simulink library "HANcoder_STM32_Target"  (R2023a)
settings: Solver=ode45  StartTime=0.0  StopTime=10.0  RelTol=1e-3  EnableMultiTasking=on
libraries: simulink x3
(part 6 of 7)

== system HANcoder_STM32_Target/Olimexino STM32/Timer Outputs/Schedule Compare Event ==
  In1 : Inport
  In2 : Inport  Port=2
  Level-2 M-file S-Function : M-S-Function  FunctionName=sfcn_timeout_scheduleevent  Parameters=tsamp
  wires:
  In1/1 -> Level-2 M-file S-Function/1
  In2/1 -> Level-2 M-file S-Function/2

== system HANcoder_STM32_Target/Olimexino STM32/UART/UART init ==
  Level-2 M-file S-Function : M-S-Function  FunctionName=sfcn_uart_init
  Term1 : Terminator
  wires:
  Level-2 M-file S-Function/1 -> Term1/1

== system HANcoder_STM32_Target/Olimexino STM32/UART/UART receive ==
  Level-2 M-file S-Function : M-S-Function  FunctionName=sfcn_uart_receive  Parameters=tsamp
  Term1 : Terminator
  Out1 : Outport
  wires:
  Level-2 M-file S-Function/2 -> Term1/1
  Level-2 M-file S-Function/1 -> Out1/1

== system HANcoder_STM32_Target/Olimexino STM32/UART/UART receive buffer status ==
  Level-2 M-file S-Function : M-S-Function  FunctionName=sfcn_uart_receive_size  Parameters=tsamp
  Out1 : Outport
  wires:
  Level-2 M-file S-Function/1 -> Out1/1

== system HANcoder_STM32_Target/Olimexino STM32/UART/UART send ==
  In1 : Inport
  Level-2 M-file S-Function : M-S-Function  FunctionName=sfcn_uart_send  Parameters=tsamp
  Term1 : Terminator
  wires:
  In1/1 -> Level-2 M-file S-Function/1
  Level-2 M-file S-Function/1 -> Term1/1

== system HANcoder_STM32_Target/Olimexino STM32/UDS/UDS Get Key ==
  S-Function : M-S-Function  FunctionName=sfcn_uds_get_key  Parameters=tsamp
  Out1 : Outport
  wires:
  S-Function/1 -> Out1/1

== system HANcoder_STM32_Target/Olimexino STM32/UDS/UDS Get Seed ==
  S-Function : M-S-Function  FunctionName=sfcn_uds_get_seed  Parameters=tsamp
  Out1 : Outport
  wires:
  S-Function/1 -> Out1/1

== system HANcoder_STM32_Target/Olimexino STM32/UDS/UDS Get Seed Event ==
  S-Function : S-Function  FunctionName=sfcn_uds_get_seed_event  SFunctionDeploymentMode=off  EnableBusSupport=off
  Out1 : Outport
  wires:
  S-Function/1 -> Out1/1

== system HANcoder_STM32_Target/Olimexino STM32/UDS/UDS Init ==
  S-Function : M-S-Function  FunctionName=sfcn_uds_init

== system HANcoder_STM32_Target/Olimexino STM32/UDS/UDS Set Key Verfied ==
  In1 : Inport
  S-Function : M-S-Function  FunctionName=sfcn_uds_set_key_verified  Parameters=tsamp
  wires:
  In1/1 -> S-Function/1

== system HANcoder_STM32_Target/Olimexino STM32/UDS/UDS Set Seed ==
  In1 : Inport
  S-Function : M-S-Function  FunctionName=sfcn_uds_set_seed  Parameters=tsamp
  wires:
  In1/1 -> S-Function/1

== system HANcoder_STM32_Target/Olimexino STM32/UDS/UDS Verify Key Event ==
  S-Function : S-Function  FunctionName=sfcn_uds_verify_key_event  SFunctionDeploymentMode=off  EnableBusSupport=off
  Out1 : Outport
  wires:
  S-Function/1 -> Out1/1

== system HANcoder_STM32_Target/STM32-E407/Analog Inputs/Analog Input ==
  Level-2 M-file S-Function : M-S-Function  FunctionName=sfcn_analog_in  Parameters=tsamp, pinID
  Out1 : Outport
  wires:
  Level-2 M-file S-Function/1 -> Out1/1

== system HANcoder_STM32_Target/STM32-E407/Analog Outputs/Analog Output ==
  In1 : Inport
  Data Type Conversion : DataTypeConversion  OutDataTypeStr=uint16  SaturateOnIntegerOverflow=off  RndMeth=Floor
  Level-2 M-file S-Function : M-S-Function  FunctionName=sfcn_analog_out  Parameters=tsamp, pinID
  Saturation : Saturate  UpperLimit=4095  LowerLimit=0
  wires:
  Saturation/1 -> Level-2 M-file S-Function/1
  Data Type Conversion/1 -> Saturation/1
  In1/1 -> Data Type Conversion/1

== system HANcoder_STM32_Target/STM32-E407/CAN/CAN ==
  CAN receive : Subsystem  Tag=HANcoder_TARGET_STM32_E407  mask(CAN receive){canBus=CAN 1, outputNumber=1, dataType=uint8, byteOrder=off, tsamp=-1}
      mask prompts: canBus "CAN channel"; outputNumber "Output ports"; dataType "Output datatype"; byteOrder "Byte order: Checked = MSB first, unchecked = LSB first."; tsamp "Sample time"
      mask help:
      | Function
      | ==========
      | Receive the newest message from the specified CAN channel.
      |
      | Parameters
      | ==========
      | CAN channel:             The CAN channel to send the message on.
      | Output ports:             The amount of output ports
      | Output datatype:       The datatype of the output ports
      | Byte order:                 Select MSB or LSB first
      | Sample time:              -1 or divisible by base sample time [seconds]
      |
      | Input
      | ==========
      | Port 1:                       CAN ID(uint32) in hexadecimal ie: hex2dec('0a')
      |
      | Output
      | ==========
      | Port 1:                       Checks for new message(int8)
      | Port 2..9                     Message data
      mask init:
      | sfcn_can_receive_mcb(canBus, outputNumber, dataType, byteOrder)
      settings: MoveFcn=drawLogos
      mask Help: web('sfcn_can_receive.html');
      mask TypeOptions canBus: CAN 1 | CAN 2
      mask TypeOptions dataType: int8 | uint8 | int16 | uint16 | int32 | uint32 | boolean
      mask Display:
      | fprintf('Receive on\nCAN %x', canBus);
      | port_label('output', 1, 'new');
      | port_label('input', 1, 'ID');patch([75 81 81],[8 14 2],[1 0 0]);patch([83 83 89],[14 2 8],[0 0 0.35]);
  CAN receive packed : Subsystem  Tag=HANcoder_TARGET_STM32_E407  mask(CAN receive packed){canBus=CAN 1, canID=hex2dec('80'), tsamp=-1}
      mask prompts: canBus "CAN channel"; canID "Can ID (in hex)"; tsamp "Sample time"
      mask help:
      | Function
      | ==========
      | Receive the newest message from the specified CAN channel, packed in a CAN message signal.
      | The first output checks the receiving of new data.
      |
      | CAN channel: The specified CAN channel will be used to receive the message on.
      |
      | CAN ID (in hex): Only the message with the specified CAN identifier (ID) is received. The ID is written in hexadecimal format, ie: hex2dec('0A')
      |
      | PS. No data is unpacked by the 'CAN Unpack' block when the data output is directly connected to a terminator (an example, placing a *1 'Gain' in between will solve this).
      mask init:
      | sfcn_can_receive_packed_mcb(canBus, canID)
      settings: MoveFcn=drawLogos
      mask Help: web('sfcn_can_receive_packed.html');
      mask TypeOptions canBus: CAN 1 | CAN 2
      mask Display: fprintf('Receive packed CAN\nmessage on CAN %x\nID %xh', canBus, canID);patch([95 101 101],[8 14 2],[1 0 0]);patch([103 103 109],[14 2 8],[0 0 0.35]);
  CAN send : Subsystem  Tag=HANcoder_TARGET_STM32_E407  mask(CAN send){canBus=CAN 1, frameType=Standard (11 bit), inputNumber=8, dataType=uint8, byteOrder=on, tsamp=-1}
      mask prompts: canBus "CAN channel"; frameType "Identifier type"; inputNumber "Input ports"; dataType "Input datatype"; byteOrder "Byte order: Checked = MSB first, unchecked = LSB first."; tsamp "Sample time"
      mask help:
      | Function
      | ==========
      | Send a message on the CAN channel.
      |
      | Parameters
      | ==========
      | CAN channel:           The CAN channel to send the message on.
      | Identifier type:         normal or extended ID's
      | Input ports:              The amount of input ports
      | Input datatype:        The datatype of the input ports
      | Byte order:               Select MSB or LSB first
      | Sample time:            -1 or divisible by base sample time [seconds]
      |
      | Input
      | ==========
      | Port 1:                   CAN ID(uint32) in hexadecimal ie: hex2dec('0a')
      | Port 2..9                CAN message data
      mask init:
      | sfcn_can_send_mcb(canBus, frameType, inputNumber, dataType, byteOrder)
      settings: MoveFcn=drawLogos
      mask Help: web('sfcn_can_send.html');
      mask TypeOptions canBus: CAN 1 | CAN 2
      mask TypeOptions frameType: Standard (11 bit) | Extended (29 bit)
      mask TypeOptions dataType: int8 | uint8 | int16 | uint16 | int32 | uint32 | boolean
      mask Display:
      | fprintf('Send on\nCAN %x', canBus);
      | port_label('input', 1, 'ID');patch([65 71 71],[8 14 2],[1 0 0]);patch([73 73 79],[14 2 8],[0 0 0.35]);
  CAN send packed : Subsystem  Tag=HANcoder_TARGET_STM32_E407  mask(CAN send packed){canBus=CAN 1, tsamp=-1}
      mask prompts: canBus "CAN channel"; tsamp "Sample time"
      mask help:
      | Function
      | ==========
      | Send a packed CAN message on the specified CAN channel.
      |
      | CAN channel: The specified CAN channel will be used to send the message on.
      |
      | The CAN ID, identifier type and formatting of the data is included in the packed CAN message.
      mask init:
      | sfcn_can_send_packed_mcb(canBus)
      settings: MoveFcn=drawLogos
      mask Help: web('sfcn_can_send_packed.html');
      mask TypeOptions canBus: CAN 1 | CAN 2
      mask Display: fprintf('Send packed CAN\n message on CAN %x', canBus);patch([95 101 101],[8 14 2],[1 0 0]);patch([103 103 109],[14 2 8],[0 0 0.35]);

== system HANcoder_STM32_Target/STM32-E407/CAN/CANopenNode ==
  CANopenNode Init : Subsystem  Tag=HANcoder_TARGET_STM32_E407  mask(CANopenNode Init){channel=CAN 1}
      mask prompts: channel "CAN channel"
      mask help:
      | Function
      | ==========
      | Initializes the CANopenNode stack for the particular CAN channel.
      |
      | CAN channel: The specified CAN channel will be used by the communication stack.
      mask init:
      | sfcn_can_canopennode_init_mcb(channel)
      settings: MoveFcn=drawLogos
      mask Help: web('sfcn_can_canopennode_init.html');
      mask TypeOptions channel: CAN 1 | CAN 2
      mask Display: fprintf('CANopenNode\n Init on CAN %d', channel);patch([95 101 101],[8 14 2],[1 0 0]);patch([103 103 109],[14 2 8],[0 0 0.35]);
  CANopenNode OD Read : Subsystem  Tag=HANcoder_TARGET_STM32_E407  mask(CANopenNode OD Read){index=hex2dec('6200'), subIndex=1, dataType=uint8, tsamp=-1}
      mask prompts: index "OD index"; subIndex "OD subindex"; dataType "OD data type"; tsamp "Sample time"
      mask help:
      | Function
      | ==========
      | Reads a data value from the internal object dictionary.
      |
      | OD Index: Index of the object dictionary to read from.
      | OD Subindex: Subindex of the object dictionary to read from.
      | OD Data type: Data type of the object dictionary to read from.
      mask init:
      | sfcn_can_canopennode_od_read_mcb(index, subIndex, dataType)
      settings: MoveFcn=drawLogos
      mask Help: web('sfcn_can_canopennode_od_read.html');
      mask TypeOptions dataType: int8 | uint8 | int16 | uint16 | int32 | uint32
      mask Display: fprintf('CANopenNode\n OD Read\nindex: 0x%x\nsubindex: %d', index, subIndex');patch([95 101 101],[8 14 2],[1 0 0]);patch([103 103 109],[14 2 8],[0 0 0.35]);
  CANopenNode OD Write : Subsystem  Tag=HANcoder_TARGET_STM32_E407  mask(CANopenNode OD Write){index=hex2dec('6000'), subIndex=1, dataType=uint8, tsamp=-1}
      mask prompts: index "OD index"; subIndex "OD subindex"; dataType "OD data type"; tsamp "Sample time"
      mask help:
      | Function
      | ==========
      | Writes a data value to the internal object dictionary.
      |
      | OD Index: Index of the object dictionary to write to.
      | OD Subindex: Subindex of the object dictionary to write to.
      | OD Data type: Data type of the object dictionary to write to.
      mask init:
      | sfcn_can_canopennode_od_write_mcb(index, subIndex, dataType)
      settings: MoveFcn=drawLogos
      mask Help: web('sfcn_can_canopennode_od_write.html');
      mask TypeOptions dataType: int8 | uint8 | int16 | uint16 | int32 | uint32
      mask Display: fprintf('CANopenNode\n OD Write\nindex: 0x%x\nsubindex: %d', index, subIndex);patch([95 101 101],[8 14 2],[1 0 0]);patch([103 103 109],[14 2 8],[0 0 0.35]);

== system HANcoder_STM32_Target/STM32-E407/Digital Inputs/Digital Input ==
  Level-2 M-file S-Function : M-S-Function  FunctionName=sfcn_digital_in  Parameters=tsamp, pinID, config
  Out1 : Outport
  wires:
  Level-2 M-file S-Function/1 -> Out1/1

== system HANcoder_STM32_Target/STM32-E407/Digital Outputs/Digital Output ==
  In1 : Inport
  Level-2 M-file S-Function : M-S-Function  FunctionName=sfcn_digital_out  Parameters=tsamp, pinID, config
  wires:
  In1/1 -> Level-2 M-file S-Function/1

== system HANcoder_STM32_Target/STM32-E407/Error Handling/Clear errors ==
  Trigger : TriggerPort  VariantControl=(inherit)
  Level-2 M-file S-Function : M-S-Function  FunctionName=sfcn_controller_error_clearerrors  Parameters=eepromString

== system HANcoder_STM32_Target/STM32-E407/Error Handling/Delete error ==
  Trigger : TriggerPort  VariantControl=(inherit)
  Constant : Constant  OutDataTypeStr=uint8  SampleTime=-1
  Gnd1 : Ground
  Gnd2 : Ground
  Level-2 M-file S-Function : M-S-Function  FunctionName=sfcn_controller_error_deleteerror_in  Parameters=useInPorts, errorID, para
  wires:
  Constant/1 -> Level-2 M-file S-Function/3
  Gnd1/1 -> Level-2 M-file S-Function/1
  Gnd2/1 -> Level-2 M-file S-Function/2

== system HANcoder_STM32_Target/STM32-E407/Error Handling/Read active error ==
  In1 : Inport
  Level-2 M-file S-Function : M-S-Function  FunctionName=sfcn_controller_error_readerror  Parameters=tsamp
  numbers : Outport
  code : Outport  Port=2
  parameter : Outport  Port=3
  Xtimes : Outport  Port=4
  timestamp : Outport  Port=5
  wires:
  In1/1 -> Level-2 M-file S-Function/1
  Level-2 M-file S-Function/5 -> timestamp/1
  Level-2 M-file S-Function/4 -> Xtimes/1
  Level-2 M-file S-Function/3 -> parameter/1
  Level-2 M-file S-Function/2 -> code/1
  Level-2 M-file S-Function/1 -> numbers/1

== system HANcoder_STM32_Target/STM32-E407/Error Handling/Read stored error ==
  In1 : Inport
  Level-2 M-file S-Function : M-S-Function  FunctionName=sfcn_controller_error_readerror  Parameters=tsamp
  numbers : Outport
  code : Outport  Port=2
  parameter : Outport  Port=3
  Xtimes : Outport  Port=4
  timestamp : Outport  Port=5
  wires:
  Level-2 M-file S-Function/1 -> numbers/1
  Level-2 M-file S-Function/2 -> code/1
  Level-2 M-file S-Function/3 -> parameter/1
  Level-2 M-file S-Function/4 -> Xtimes/1
  Level-2 M-file S-Function/5 -> timestamp/1
  In1/1 -> Level-2 M-file S-Function/1

== system HANcoder_STM32_Target/STM32-E407/Error Handling/Search active error ==
  In1 : Inport
  In2 : Inport  Port=2
  Level-2 M-file S-Function : M-S-Function  FunctionName=sfcn_controller_error_searcherror  Parameters=tsamp
  occurrence : Outport
  timestamp : Outport  Port=2
  wires:
  Level-2 M-file S-Function/2 -> timestamp/1
  Level-2 M-file S-Function/1 -> occurrence/1
  In2/1 -> Level-2 M-file S-Function/2
  In1/1 -> Level-2 M-file S-Function/1

== system HANcoder_STM32_Target/STM32-E407/Error Handling/Search stored error ==
  In1 : Inport
  In2 : Inport  Port=2
  Level-2 M-file S-Function : M-S-Function  FunctionName=sfcn_controller_error_searcherror  Parameters=tsamp
  occurrence : Outport
  timestamp : Outport  Port=2
  wires:
  In1/1 -> Level-2 M-file S-Function/1
  In2/1 -> Level-2 M-file S-Function/2
  Level-2 M-file S-Function/1 -> occurrence/1
  Level-2 M-file S-Function/2 -> timestamp/1

== system HANcoder_STM32_Target/STM32-E407/Error Handling/Store error  ==
  Trigger : TriggerPort  VariantControl=(inherit)
  Gnd1 : Ground
  Gnd2 : Ground
  Level-2 M-file S-Function : M-S-Function  FunctionName=sfcn_controller_error_storeerror_in  Parameters=useInPorts, errorCode, parameter
  wires:
  Gnd2/1 -> Level-2 M-file S-Function/2
  Gnd1/1 -> Level-2 M-file S-Function/1

== system HANcoder_STM32_Target/STM32-E407/Error Handling/Total Errors ==
  Level-2 M-file S-Function : M-S-Function  FunctionName=sfcn_controller_error_totalerrors  Parameters=eepromString, tsamp
  Out1 : Outport
  Out2 : Outport  Port=2
  wires:
  Level-2 M-file S-Function/2 -> Out2/1
  Level-2 M-file S-Function/1 -> Out1/1

== system HANcoder_STM32_Target/STM32-E407/File Logger/File Logger Close ==
  Trigger : TriggerPort  VariantControl=(inherit)
  Level-2 M-file S-Function : M-S-Function  FunctionName=sfcn_filelogger_close

== system HANcoder_STM32_Target/STM32-E407/File Logger/File Logger Init ==
  (Re)start : TriggerPort  VariantControl=(inherit)
  Level-2 M-file S-Function : M-S-Function  FunctionName=sfcn_filelogger_init

== system HANcoder_STM32_Target/STM32-E407/File Logger/File Logger Signal ==
  In1 : Inport
  Level-2 M-file S-Function : M-S-Function  FunctionName=sfcn_filelogger_signal  Parameters=dataType
  wires:
  In1/1 -> Level-2 M-file S-Function/1

== system HANcoder_STM32_Target/STM32-E407/Memory/EEPROM ==
  Erase EEPROM : Subsystem  Tag=HANcoder_TARGET_STM32_E407  mask(Erase EEPROM){}
      mask help:
      | Function
      | ========
      | Erases all identifier values from EEPROM.
      |
      | Triggerport
      | ===========
      | Connect the port to a trigger source to execute the block only when necessary.
      mask init:
      | sfcn_eeprom_clear_mcb();
      settings: MoveFcn=drawLogos
      mask Display: fprintf('Erase EEPROM');patch([80 86 86],[8 14 2],[1 0 0]);patch([88 88 94],[14 2 8],[0 0 0.35]);
  Read from EEPROM : Subsystem  Tag=HANcoder_TARGET_STM32_E407  mask(Read from EEPROM){tsamp=-1}
      mask prompts: tsamp "Sample time"
      mask help:
      | Function
      | ========
      | Read a value from the specified EEPROM identifier.
      |
      | Inport
      | ==========
      | id:
      |   The EEPROM identifier. This input is of type UINT8 and can have a value
      |   between 0..255 to select one of the 256 supported application specific
      |   identifiers.
      |
      | Outport
      | =======
      | value:
      |   The value read from the EEPROM identifier. This output is of type UINT16.
      mask init:
      | sfcn_eeprom_read_mcb();
      settings: MoveFcn=drawLogos
      mask Display:
      | fprintf('Read from EEPROM');
      | port_label('input', 1, 'id');
      | port_label('output', 1, 'value');patch([150 156 156],[8 14 2],[1 0 0]);patch([158 158 164],[14 2 8],[0 0 0.35]);
  Save EEPROM : Subsystem  Tag=HANcoder_TARGET_STM32_E407  mask(Save EEPROM){}
      mask help:
      | Function
      | ========
      | The STM32 controller does not have dedicated EEPROM on-chip. All EEPROM
      | write, read and erase operations are therefore performed in a RAM buffer.
      | To make sure RAM buffer contents are still valid after a power-off, its
      | contents needs to be save in flash EEPROM, which is achieved with this
      | block. This is typically called during the software shutdown sequence,
      | right before power off.
      |
      | Triggerport
      | ===========
      | Connect the port to a trigger source to execute the block only when necessary.
      mask init:
      | sfcn_eeprom_save_mcb();
      settings: MoveFcn=drawLogos
      mask Display: fprintf('Save EEPROM');patch([80 86 86],[8 14 2],[1 0 0]);patch([88 88 94],[14 2 8],[0 0 0.35]);
  Write to EEPROM : Subsystem  Tag=HANcoder_TARGET_STM32_E407  mask(Write to EEPROM){tsamp=-1}
      mask prompts: tsamp "Sample time"
      mask help:
      | Function
      | ========
      | Write the value to the specified EEPROM identifier.
      |
      | Inport
      | ==========
      | id:
      |   The EEPROM identifier. This input is of type UINT8 and can have a value
      |   between 0..255 to select one of the 256 supported application specific
      |   identifiers.
      | value:
      |   The value to write to the EEPROM identifier. This input is of type UINT16.
      mask init:
      | sfcn_eeprom_write_mcb();
      settings: MoveFcn=drawLogos
      mask Display:
      | fprintf('Write to EEPROM');
      | port_label('input', 1, 'id');
      | port_label('input', 2, 'value');patch([150 156 156],[8 14 2],[1 0 0]);patch([158 158 164],[14 2 8],[0 0 0.35]);

== system HANcoder_STM32_Target/STM32-E407/PWM Outputs/PWM Duty Cycle ==
  In1 : Inport
  Level-2 M-file S-Function : M-S-Function  FunctionName=sfcn_pwmout_setduty  Parameters=tsamp
  wires:
  In1/1 -> Level-2 M-file S-Function/1

== system HANcoder_STM32_Target/STM32-E407/PWM Outputs/PWM Init ==
  S-Function : S-Function  FunctionName=sfcn_pwmout_init  SFunctionDeploymentMode=off  EnableBusSupport=off
  Term1 : Terminator
  wires:
  S-Function/1 -> Term1/1

== system HANcoder_STM32_Target/STM32-E407/Real-time Clock/Get Real-time Clock ==
  Level-2 M-file S-Function : M-S-Function  FunctionName=sfcn_get_rtc  Parameters=tsamp
  WeekDay : Outport
  Date : Outport  Port=2
  Month : Outport  Port=3
  Year : Outport  Port=4
  Hours : Outport  Port=5
  Minutes : Outport  Port=6
  Seconds : Outport  Port=7
  wires:
  Level-2 M-file S-Function/3 -> Month/1
  Level-2 M-file S-Function/6 -> Minutes/1
  Level-2 M-file S-Function/5 -> Hours/1
  Level-2 M-file S-Function/4 -> Year/1
  Level-2 M-file S-Function/1 -> WeekDay/1
  Level-2 M-file S-Function/7 -> Seconds/1
  Level-2 M-file S-Function/2 -> Date/1

== system HANcoder_STM32_Target/STM32-E407/Real-time Clock/Set Real-time Clock ==
  WeekDay : Inport
  Date : Inport  Port=2
  Month : Inport  Port=3
  Year : Inport  Port=4
  Hours : Inport  Port=5
  Minutes : Inport  Port=6
  Seconds : Inport  Port=7
  Trigger : TriggerPort  VariantControl=(inherit)  PortDimensions=1
  Level-2 M-file S-Function : M-S-Function  FunctionName=sfcn_set_rtc
  wires:
  WeekDay/1 -> Level-2 M-file S-Function/1
  Date/1 -> Level-2 M-file S-Function/2
  Month/1 -> Level-2 M-file S-Function/3
  Year/1 -> Level-2 M-file S-Function/4
  Hours/1 -> Level-2 M-file S-Function/5
  Minutes/1 -> Level-2 M-file S-Function/6
  Seconds/1 -> Level-2 M-file S-Function/7

== system HANcoder_STM32_Target/STM32-E407/SPI/SPI master init ==
  Level-2 M-file S-Function : M-S-Function  FunctionName=sfcn_spi_master_init

== system HANcoder_STM32_Target/STM32-E407/SPI/SPI master transfer ==
  In1 : Inport
  Level-2 M-file S-Function : M-S-Function  FunctionName=sfcn_spi_master_transfer  Parameters=tsamp
  Out1 : Outport
  wires:
  Level-2 M-file S-Function/1 -> Out1/1
  In1/1 -> Level-2 M-file S-Function/1

== system HANcoder_STM32_Target/STM32-E407/System Config/Base Sample Time config ==
  note: This constant and terminator block introduces the base sample time,
      | set in Base Sample Time config block, to the model. Blocks  with inherited [-1]
      | sample time wich are not connected to blocks with specifically set sample times
      | will use this value. This block also sets the fixed step time parameter in the Simulink Solver.
      | This works during initialization of simulation or build.
  Level-2 M-file S-Function : M-S-Function  FunctionName=sfcn_base_sample_time  Parameters=baseSampleTime, extraStack
  SampleTimeCrowBar : Constant  InitFcn=|  VectorParams1D=off  OutDataTypeStr=boolean  SampleTime=0.01
      | SampleTimeMiliSeconds = get_param(find_system(bdroot, 'LookUnderMasks', 'all', 'FollowLinks', 'off',  'Name', 'Base Sample Time config'), 'baseSampleTime');
      |                                                                                                                                                             
      | SampleTimeSeconds = str2num(SampleTimeMiliSeconds{1,1})/1000;                                                                                               
      |                                                                                                                                                             
      | set_param(bdroot, 'FixedStep', num2str(SampleTimeSeconds));                                                                                                 
      |                                                                                                                                                             
      | set_param(gcb, 'SampleTime', num2str(get_param(bdroot, 'FixedStep')));                                                                                      
      | clear SampleTimeSeconds SampleTimeMiliSeconds
  Terminator : Terminator
  wires:
  SampleTimeCrowBar/1 -> Terminator/1

== system HANcoder_STM32_Target/STM32-E407/System Config/Build settings ==

== system HANcoder_STM32_Target/STM32-E407/System Config/CAN config ==
  Level-2 M-file S-Function : M-S-Function  FunctionName=sfcn_can_config

== system HANcoder_STM32_Target/STM32-E407/System Config/Custom ID config ==
  Level-2 M-file S-Function : M-S-Function  RequirementInfo={}  FunctionName=sfcn_custom_version_config  Parameters=softID

== system HANcoder_STM32_Target/STM32-E407/System Config/Ethernet config ==
  Level-2 M-file S-Function : M-S-Function  FunctionName=sfcn_ethernet_config

== system HANcoder_STM32_Target/STM32-E407/System Config/FTP server config ==
  Level-2 M-file S-Function : M-S-Function  FunctionName=sfcn_ftp_server_config

== system HANcoder_STM32_Target/STM32-E407/System Config/XCP on CAN config ==
  Level-2 M-file S-Function : M-S-Function  RequirementInfo={} %GIDa_75ebdf1d_e085_4bd4_9cf7_36846954f0a6  FunctionName=sfcn_can_xcp_config  Parameters=canBus, croID, dtoID

== system HANcoder_STM32_Target/STM32-E407/System Config/XCP on TCP//IP config ==
  Level-2 M-file S-Function : M-S-Function  RequirementInfo={} %GIDa_75ebdf1d_e085_4bd4_9cf7_36846954f0a6  FunctionName=sfcn_tcpip_xcp_config  Parameters=port

== system HANcoder_STM32_Target/STM32-E407/System Config/XCP on USB config ==
  Level-2 M-file S-Function : M-S-Function  RequirementInfo={} %GIDa_75ebdf1d_e085_4bd4_9cf7_36846954f0a6  FunctionName=sfcn_usb_xcp_config

== system HANcoder_STM32_Target/STM32-E407/System Management/Enter Critical Section ==
  Level-2 M-file S-Function : M-S-Function  FunctionName=sfcn_critical_enter  Parameters=tsamp

== system HANcoder_STM32_Target/STM32-E407/System Management/Exit Critical Section ==
  Level-2 M-file S-Function : M-S-Function  FunctionName=sfcn_critical_exit  Parameters=tsamp

== system HANcoder_STM32_Target/STM32-E407/System Management/Get CPU load ==
  Level-2 M-file S-Function : M-S-Function  FunctionName=sfcn_controller_cpu_getload  Parameters=tsamp, mode
  Out1 : Outport
  wires:
  Level-2 M-file S-Function/1 -> Out1/1

== system HANcoder_STM32_Target/STM32-E407/System Management/Get free Heap ==
  Level-2 M-file S-Function : M-S-Function  FunctionName=sfcn_controller_getheap  Parameters=tsamp
  Out1 : Outport
  wires:
  Level-2 M-file S-Function/1 -> Out1/1

== system HANcoder_STM32_Target/STM32-E407/System Management/Get free Stack ==
  Level-2 M-file S-Function : M-S-Function  FunctionName=sfcn_controller_getstack  Parameters=tsamp, taskIdx
  Out1 : Outport
  wires:
  Level-2 M-file S-Function/1 -> Out1/1

== system HANcoder_STM32_Target/STM32-E407/System Management/Reset ECU ==
  Trigger : TriggerPort  VariantControl=(inherit)
  Level-2 M-file S-Function : M-S-Function  FunctionName=sfcn_controller_reset

== system HANcoder_STM32_Target/STM32-E407/Timer Inputs/Quadrature Encoder Get ==
  Data Type Conversion : DataTypeConversion  OutDataTypeStr=boolean  SaturateOnIntegerOverflow=off  RndMeth=Floor
  Detect Increase : simulink/Logic and Bit Operations/Detect Increase  vinit=0.0  OutDataTypeStr=uint8
  Gnd1 : Ground
  Level-2 M-file S-Function : M-S-Function  FunctionName=sfcn_quad_encoder_get  Parameters=tsamp, moduleID
  Out1 : Outport
  wires:
  Data Type Conversion/1 -> Level-2 M-file S-Function/1
  Detect Increase/1 -> Data Type Conversion/1
  Gnd1/1 -> Detect Increase/1
  Level-2 M-file S-Function/1 -> Out1/1

== system HANcoder_STM32_Target/STM32-E407/Timer Inputs/Timer Input Get ==
  Level-2 M-file S-Function : M-S-Function  FunctionName=sfcn_timein_get  Parameters=tsamp
  Out1 : Outport
  Out2 : Outport  Port=2
  Out3 : Outport  Port=3
  Out4 : Outport  Port=4
  Out5 : Outport  Port=5
  Out6 : Outport  Port=6
  Out7 : Outport  Port=7
  wires:
  Level-2 M-file S-Function/5 -> Out5/1
  Level-2 M-file S-Function/4 -> Out4/1
  Level-2 M-file S-Function/3 -> Out3/1
  Level-2 M-file S-Function/2 -> Out2/1
  Level-2 M-file S-Function/1 -> Out1/1
  Level-2 M-file S-Function/6 -> Out6/1
  Level-2 M-file S-Function/7 -> Out7/1

== system HANcoder_STM32_Target/STM32-E407/Timer Inputs/Timer Input IRQ ==
  S-Function : S-Function  FunctionName=sfcn_timein_irq  SFunctionDeploymentMode=off  EnableBusSupport=off
  Out1 : Outport
  wires:
  S-Function/1 -> Out1/1

== system HANcoder_STM32_Target/STM32-E407/Timer Outputs/Compare Event IRQ ==
  S-Function : S-Function  FunctionName=sfcn_timeout_event_irq  SFunctionDeploymentMode=off  EnableBusSupport=off
  Out1 : Outport
  wires:
  S-Function/1 -> Out1/1

== system HANcoder_STM32_Target/STM32-E407/Timer Outputs/Get Free Running Counter ==
  Level-2 M-file S-Function : M-S-Function  FunctionName=sfcn_timeout_getrunningcounter  Parameters=tsamp
  Out1 : Outport
  wires:
  Level-2 M-file S-Function/1 -> Out1/1

== system HANcoder_STM32_Target/STM32-E407/Timer Outputs/Get Last Event Counter ==
  Level-2 M-file S-Function : M-S-Function  FunctionName=sfcn_timeout_getlasteventcounter  Parameters=tsamp
  Out1 : Outport
  wires:
  Level-2 M-file S-Function/1 -> Out1/1

== system HANcoder_STM32_Target/STM32-E407/Timer Outputs/Output Compare Init ==
  S-Function : S-Function  FunctionName=sfcn_timeout_init  SFunctionDeploymentMode=off  EnableBusSupport=off
  Term1 : Terminator
  wires:
  S-Function/1 -> Term1/1

== system HANcoder_STM32_Target/STM32-E407/Timer Outputs/Reset Free Running Counter ==
  Trigger : TriggerPort  VariantControl=(inherit)
  Level-2 M-file S-Function : M-S-Function  FunctionName=sfcn_timeout_resetcounter

== system HANcoder_STM32_Target/STM32-E407/Timer Outputs/Schedule Compare Event ==
  In1 : Inport
  In2 : Inport  Port=2
  Level-2 M-file S-Function : M-S-Function  FunctionName=sfcn_timeout_scheduleevent  Parameters=tsamp
  wires:
  In1/1 -> Level-2 M-file S-Function/1
  In2/1 -> Level-2 M-file S-Function/2

== system HANcoder_STM32_Target/STM32-E407/UART/UART init ==
  Level-2 M-file S-Function : M-S-Function  FunctionName=sfcn_uart_init
  Term1 : Terminator
  wires:
  Level-2 M-file S-Function/1 -> Term1/1

== system HANcoder_STM32_Target/STM32-E407/UART/UART receive ==
  Level-2 M-file S-Function : M-S-Function  FunctionName=sfcn_uart_receive  Parameters=tsamp
  Term1 : Terminator
  Out1 : Outport
  wires:
  Level-2 M-file S-Function/1 -> Out1/1
  Level-2 M-file S-Function/2 -> Term1/1

== system HANcoder_STM32_Target/STM32-E407/UART/UART receive buffer status ==
  Level-2 M-file S-Function : M-S-Function  FunctionName=sfcn_uart_receive_size  Parameters=tsamp
  Out1 : Outport
  wires:
  Level-2 M-file S-Function/1 -> Out1/1

== system HANcoder_STM32_Target/STM32-E407/UART/UART send ==
  In1 : Inport
  Level-2 M-file S-Function : M-S-Function  FunctionName=sfcn_uart_send  Parameters=tsamp
  Term1 : Terminator
  wires:
  Level-2 M-file S-Function/1 -> Term1/1
  In1/1 -> Level-2 M-file S-Function/1

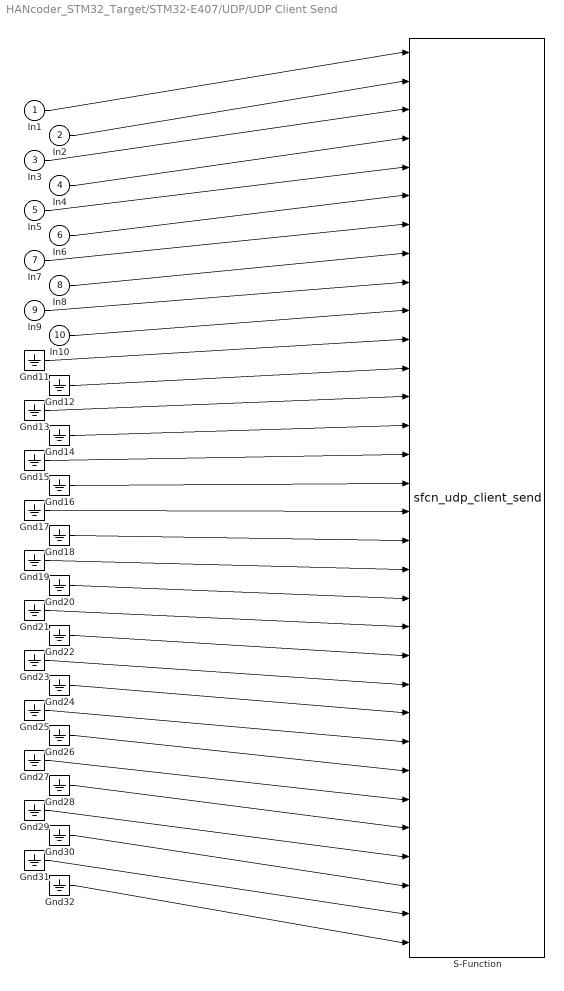
== system HANcoder_STM32_Target/STM32-E407/UDP/UDP Client Send ==
  In1 : Inport
  In2 : Inport  Port=2
  In3 : Inport  Port=3
  In4 : Inport  Port=4
  In5 : Inport  Port=5
  In6 : Inport  Port=6
  In7 : Inport  Port=7
  In8 : Inport  Port=8
  In9 : Inport  Port=9
  In10 : Inport  Port=10
  Gnd{11..32} (22 alike) : Ground
  S-Function : M-S-Function  FunctionName=sfcn_udp_client_send  Parameters=tsamp, dataType
  wires:
  In1/1 -> S-Function/1
  In2/1 -> S-Function/2
  In3/1 -> S-Function/3
  In4/1 -> S-Function/4
  In5/1 -> S-Function/5
  In6/1 -> S-Function/6
  In7/1 -> S-Function/7
  In8/1 -> S-Function/8
  In9/1 -> S-Function/9
  In10/1 -> S-Function/10
  Gnd11/1 -> S-Function/11
  Gnd12/1 -> S-Function/12
  Gnd13/1 -> S-Function/13
  Gnd14/1 -> S-Function/14
  Gnd15/1 -> S-Function/15
  Gnd16/1 -> S-Function/16
  Gnd17/1 -> S-Function/17
  Gnd18/1 -> S-Function/18
  Gnd19/1 -> S-Function/19
  Gnd20/1 -> S-Function/20
  Gnd21/1 -> S-Function/21
  Gnd22/1 -> S-Function/22
  Gnd23/1 -> S-Function/23
  Gnd24/1 -> S-Function/24
  Gnd25/1 -> S-Function/25
  Gnd26/1 -> S-Function/26
  Gnd27/1 -> S-Function/27
  Gnd28/1 -> S-Function/28
  Gnd29/1 -> S-Function/29
  Gnd30/1 -> S-Function/30
  Gnd31/1 -> S-Function/31
  Gnd32/1 -> S-Function/32

== system HANcoder_STM32_Target/STM32-E407/UDP/UDP Server Init ==
  S-Function : M-S-Function  FunctionName=sfcn_udp_server_init

== system HANcoder_STM32_Target/STM32-E407/UDP/UDP Server New Data Available ==
  S-Function : M-S-Function  FunctionName=sfcn_udp_server_new  Parameters=tsamp
  Out1 : Outport
  wires:
  S-Function/1 -> Out1/1

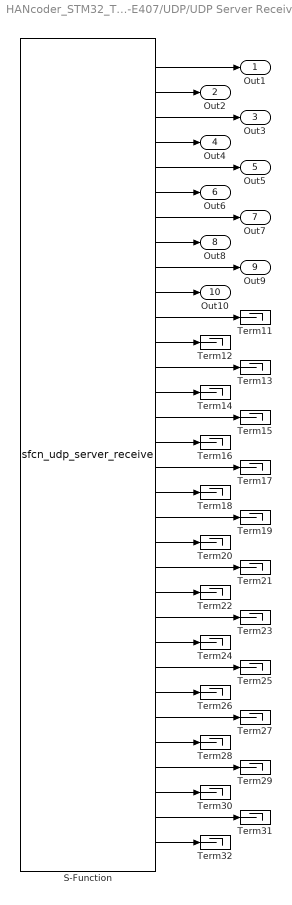
== system HANcoder_STM32_Target/STM32-E407/UDP/UDP Server Receive ==
  S-Function : M-S-Function  FunctionName=sfcn_udp_server_receive  Parameters=tsamp, dataType
  Term{11..32} (22 alike) : Terminator
  Out1 : Outport
  Out2 : Outport  Port=2
  Out3 : Outport  Port=3
  Out4 : Outport  Port=4
  Out5 : Outport  Port=5
  Out6 : Outport  Port=6
  Out7 : Outport  Port=7
  Out8 : Outport  Port=8
  Out9 : Outport  Port=9
  Out10 : Outport  Port=10
  wires:
  S-Function/1 -> Out1/1
  S-Function/2 -> Out2/1
  S-Function/3 -> Out3/1
  S-Function/4 -> Out4/1
  S-Function/5 -> Out5/1
  S-Function/6 -> Out6/1
  S-Function/7 -> Out7/1
  S-Function/8 -> Out8/1
  S-Function/9 -> Out9/1
  S-Function/10 -> Out10/1
  S-Function/11 -> Term11/1
  S-Function/12 -> Term12/1
  S-Function/13 -> Term13/1
  S-Function/14 -> Term14/1
  S-Function/15 -> Term15/1
  S-Function/16 -> Term16/1
  S-Function/17 -> Term17/1
  S-Function/18 -> Term18/1
  S-Function/19 -> Term19/1
  S-Function/20 -> Term20/1
  S-Function/21 -> Term21/1
  S-Function/22 -> Term22/1
  S-Function/23 -> Term23/1
  S-Function/24 -> Term24/1
  S-Function/25 -> Term25/1
  S-Function/26 -> Term26/1
  S-Function/27 -> Term27/1
  S-Function/28 -> Term28/1
  S-Function/29 -> Term29/1
  S-Function/30 -> Term30/1
  S-Function/31 -> Term31/1
  S-Function/32 -> Term32/1

== system HANcoder_STM32_Target/STM32-E407/UDP/UDP Server Receive Size ==
  S-Function : M-S-Function  FunctionName=sfcn_udp_server_count  Parameters=tsamp
  Out1 : Outport
  wires:
  S-Function/1 -> Out1/1

== system HANcoder_STM32_Target/STM32-E407/UDS/UDS Get Key ==
  S-Function : M-S-Function  FunctionName=sfcn_uds_get_key  Parameters=tsamp
  Out1 : Outport
  wires:
  S-Function/1 -> Out1/1

== system HANcoder_STM32_Target/STM32-E407/UDS/UDS Get Seed ==
  S-Function : M-S-Function  FunctionName=sfcn_uds_get_seed  Parameters=tsamp
  Out1 : Outport
  wires:
  S-Function/1 -> Out1/1

== system HANcoder_STM32_Target/STM32-E407/UDS/UDS Get Seed Event ==
  S-Function : S-Function  FunctionName=sfcn_uds_get_seed_event  SFunctionDeploymentMode=off  EnableBusSupport=off
  Out1 : Outport
  wires:
  S-Function/1 -> Out1/1

== system HANcoder_STM32_Target/STM32-E407/UDS/UDS Init ==
  S-Function : M-S-Function  FunctionName=sfcn_uds_init

== system HANcoder_STM32_Target/STM32-E407/UDS/UDS Set Key Verfied ==
  In1 : Inport
  S-Function : M-S-Function  FunctionName=sfcn_uds_set_key_verified  Parameters=tsamp
  wires:
  In1/1 -> S-Function/1

== system HANcoder_STM32_Target/STM32-E407/UDS/UDS Set Seed ==
  In1 : Inport
  S-Function : M-S-Function  FunctionName=sfcn_uds_set_seed  Parameters=tsamp
  wires:
  In1/1 -> S-Function/1

== system HANcoder_STM32_Target/STM32-E407/UDS/UDS Verify Key Event ==
  S-Function : S-Function  FunctionName=sfcn_uds_verify_key_event  SFunctionDeploymentMode=off  EnableBusSupport=off
  Out1 : Outport
  wires:
  S-Function/1 -> Out1/1

== system HANcoder_STM32_Target/STM32-P405/Analog Inputs/Analog Input ==
  Level-2 M-file S-Function : M-S-Function  FunctionName=sfcn_analog_in  Parameters=tsamp, pinID
  Out1 : Outport
  wires:
  Level-2 M-file S-Function/1 -> Out1/1

== system HANcoder_STM32_Target/STM32-P405/CAN/CAN ==
  CAN receive : Subsystem  Tag=HANcoder_TARGET_STM32_P405  mask(CAN receive){canBus=CAN 1, outputNumber=1, dataType=uint8, byteOrder=off, tsamp=-1}
      mask prompts: canBus "CAN channel"; outputNumber "Output ports"; dataType "Output datatype"; byteOrder "Byte order: Checked = MSB first, unchecked = LSB first."; tsamp "Sample time"
      mask help:
      | Function
      | ==========
      | Receive the newest message from the specified CAN channel.
      |
      | Parameters
      | ==========
      | CAN channel:             The CAN channel to send the message on.
      | Output ports:             The amount of output ports
      | Output datatype:       The datatype of the output ports
      | Byte order:                 Select MSB or LSB first
      | Sample time:              -1 or divisible by base sample time [seconds]
      |
      | Input
      | ==========
      | Port 1:                       CAN ID(uint32) in hexadecimal ie: hex2dec('0a')
      |
      | Output
      | ==========
      | Port 1:                       Checks for new message(int8)
      | Port 2..9                     Message data
      mask init:
      | sfcn_can_receive_mcb(canBus, outputNumber, dataType, byteOrder)
      settings: MoveFcn=drawLogos
      mask Help: web('sfcn_can_receive.html');
      mask TypeOptions canBus: CAN 1 | CAN 2
      mask TypeOptions dataType: int8 | uint8 | int16 | uint16 | int32 | uint32 | boolean
      mask Display:
      | fprintf('Receive on\nCAN %x', canBus);
      | port_label('output', 1, 'new');
      | port_label('input', 1, 'ID');patch([75 81 81],[8 14 2],[1 0 0]);patch([83 83 89],[14 2 8],[0 0 0.35]);
  CAN receive packed : Subsystem  Tag=HANcoder_TARGET_STM32_P405  mask(CAN receive packed){canBus=CAN 1, canID=hex2dec('80'), tsamp=-1}
      mask prompts: canBus "CAN channel"; canID "Can ID (in hex)"; tsamp "Sample time"
      mask help:
      | Function
      | ==========
      | Receive the newest message from the specified CAN channel, packed in a CAN message signal.
      | The first output checks the receiving of new data.
      |
      | CAN channel: The specified CAN channel will be used to receive the message on.
      |
      | CAN ID (in hex): Only the message with the specified CAN identifier (ID) is received. The ID is written in hexadecimal format, ie: hex2dec('0A')
      |
      | PS. No data is unpacked by the 'CAN Unpack' block when the data output is directly connected to a terminator (an example, placing a *1 'Gain' in between will solve this).
      mask init:
      | sfcn_can_receive_packed_mcb(canBus, canID)
      settings: MoveFcn=drawLogos
      mask Help: web('sfcn_can_receive_packed.html');
      mask TypeOptions canBus: CAN 1 | CAN 2
      mask Display: fprintf('Receive packed CAN\nmessage on CAN %x\nID %xh', canBus, canID);patch([95 101 101],[8 14 2],[1 0 0]);patch([103 103 109],[14 2 8],[0 0 0.35]);
  CAN send : Subsystem  Tag=HANcoder_TARGET_STM32_P405  mask(CAN send){canBus=CAN 1, frameType=Standard (11 bit), inputNumber=8, dataType=uint8, byteOrder=on, tsamp=-1}
      mask prompts: canBus "CAN channel"; frameType "Identifier type"; inputNumber "Input ports"; dataType "Input datatype"; byteOrder "Byte order: Checked = MSB first, unchecked = LSB first."; tsamp "Sample time"
      mask help:
      | Function
      | ==========
      | Send a message on the CAN channel.
      |
      | Parameters
      | ==========
      | CAN channel:           The CAN channel to send the message on.
      | Identifier type:         normal or extended ID's
      | Input ports:              The amount of input ports
      | Input datatype:        The datatype of the input ports
      | Byte order:               Select MSB or LSB first
      | Sample time:            -1 or divisible by base sample time [seconds]
      |
      | Input
      | ==========
      | Port 1:                   CAN ID(uint32) in hexadecimal ie: hex2dec('0a')
      | Port 2..9                CAN message data
      mask init:
      | sfcn_can_send_mcb(canBus, frameType, inputNumber, dataType, byteOrder)
      settings: MoveFcn=drawLogos
      mask Help: web('sfcn_can_send.html');
      mask TypeOptions canBus: CAN 1 | CAN 2
      mask TypeOptions frameType: Standard (11 bit) | Extended (29 bit)
      mask TypeOptions dataType: int8 | uint8 | int16 | uint16 | int32 | uint32 | boolean
      mask Display:
      | fprintf('Send on\nCAN %x', canBus);
      | port_label('input', 1, 'ID');patch([65 71 71],[8 14 2],[1 0 0]);patch([73 73 79],[14 2 8],[0 0 0.35]);
  CAN send packed : Subsystem  Tag=HANcoder_TARGET_STM32_P405  mask(CAN send packed){canBus=CAN 1, tsamp=-1}
      mask prompts: canBus "CAN channel"; tsamp "Sample time"
      mask help:
      | Function
      | ==========
      | Send a packed CAN message on the specified CAN channel.
      |
      | CAN channel: The specified CAN channel will be used to send the message on.
      |
      | The CAN ID, identifier type and formatting of the data is included in the packed CAN message.
      mask init:
      | sfcn_can_send_packed_mcb(canBus)
      settings: MoveFcn=drawLogos
      mask Help: web('sfcn_can_send_packed.html');
      mask TypeOptions canBus: CAN 1 | CAN 2
      mask Display: fprintf('Send packed CAN\n message on CAN %x', canBus);patch([95 101 101],[8 14 2],[1 0 0]);patch([103 103 109],[14 2 8],[0 0 0.35]);

== system HANcoder_STM32_Target/STM32-P405/CAN/CANopenNode ==
  CANopenNode Init : Subsystem  Tag=HANcoder_TARGET_STM32_P405  mask(CANopenNode Init){channel=CAN 1}
      mask prompts: channel "CAN channel"
      mask help:
      | Function
      | ==========
      | Initializes the CANopenNode stack for the particular CAN channel.
      |
      | CAN channel: The specified CAN channel will be used by the communication stack.
      mask init:
      | sfcn_can_canopennode_init_mcb(channel)
      settings: MoveFcn=drawLogos
      mask Help: web('sfcn_can_canopennode_init.html');
      mask TypeOptions channel: CAN 1 | CAN 2
      mask Display: fprintf('CANopenNode\n Init on CAN %d', channel);patch([95 101 101],[8 14 2],[1 0 0]);patch([103 103 109],[14 2 8],[0 0 0.35]);
  CANopenNode OD Read : Subsystem  Tag=HANcoder_TARGET_STM32_P405  mask(CANopenNode OD Read){index=hex2dec('6200'), subIndex=1, dataType=uint8, tsamp=-1}
      mask prompts: index "OD index"; subIndex "OD subindex"; dataType "OD data type"; tsamp "Sample time"
      mask help:
      | Function
      | ==========
      | Reads a data value from the internal object dictionary.
      |
      | OD Index: Index of the object dictionary to read from.
      | OD Subindex: Subindex of the object dictionary to read from.
      | OD Data type: Data type of the object dictionary to read from.
      mask init:
      | sfcn_can_canopennode_od_read_mcb(index, subIndex, dataType)
      settings: MoveFcn=drawLogos
      mask Help: web('sfcn_can_canopennode_od_read.html');
      mask TypeOptions dataType: int8 | uint8 | int16 | uint16 | int32 | uint32
      mask Display: fprintf('CANopenNode\n OD Read\nindex: 0x%x\nsubindex: %d', index, subIndex');patch([95 101 101],[8 14 2],[1 0 0]);patch([103 103 109],[14 2 8],[0 0 0.35]);
  CANopenNode OD Write : Subsystem  Tag=HANcoder_TARGET_STM32_P405  mask(CANopenNode OD Write){index=hex2dec('6000'), subIndex=1, dataType=uint8, tsamp=-1}
      mask prompts: index "OD index"; subIndex "OD subindex"; dataType "OD data type"; tsamp "Sample time"
      mask help:
      | Function
      | ==========
      | Writes a data value to the internal object dictionary.
      |
      | OD Index: Index of the object dictionary to write to.
      | OD Subindex: Subindex of the object dictionary to write to.
      | OD Data type: Data type of the object dictionary to write to.
      mask init:
      | sfcn_can_canopennode_od_write_mcb(index, subIndex, dataType)
      settings: MoveFcn=drawLogos
      mask Help: web('sfcn_can_canopennode_od_write.html');
      mask TypeOptions dataType: int8 | uint8 | int16 | uint16 | int32 | uint32
      mask Display: fprintf('CANopenNode\n OD Write\nindex: 0x%x\nsubindex: %d', index, subIndex);patch([95 101 101],[8 14 2],[1 0 0]);patch([103 103 109],[14 2 8],[0 0 0.35]);

== system HANcoder_STM32_Target/STM32-P405/Digital Inputs/Digital Input ==
  Level-2 M-file S-Function : M-S-Function  FunctionName=sfcn_digital_in  Parameters=tsamp, pinID, config
  Out1 : Outport
  wires:
  Level-2 M-file S-Function/1 -> Out1/1

== system HANcoder_STM32_Target/STM32-P405/Digital Outputs/Digital Output ==
  In1 : Inport
  Level-2 M-file S-Function : M-S-Function  FunctionName=sfcn_digital_out  Parameters=tsamp, pinID, config
  wires:
  In1/1 -> Level-2 M-file S-Function/1

== system HANcoder_STM32_Target/STM32-P405/Error Handling/Clear errors ==
  Trigger : TriggerPort  VariantControl=(inherit)
  Level-2 M-file S-Function : M-S-Function  FunctionName=sfcn_controller_error_clearerrors  Parameters=eepromString

== system HANcoder_STM32_Target/STM32-P405/Error Handling/Delete error ==
  Trigger : TriggerPort  VariantControl=(inherit)
  Constant : Constant  OutDataTypeStr=uint8  SampleTime=-1
  Gnd1 : Ground
  Gnd2 : Ground
  Level-2 M-file S-Function : M-S-Function  FunctionName=sfcn_controller_error_deleteerror_in  Parameters=useInPorts, errorID, para
  wires:
  Gnd2/1 -> Level-2 M-file S-Function/2
  Gnd1/1 -> Level-2 M-file S-Function/1
  Constant/1 -> Level-2 M-file S-Function/3

== system HANcoder_STM32_Target/STM32-P405/Error Handling/Read active error ==
  In1 : Inport
  Level-2 M-file S-Function : M-S-Function  FunctionName=sfcn_controller_error_readerror  Parameters=tsamp
  numbers : Outport
  code : Outport  Port=2
  parameter : Outport  Port=3
  Xtimes : Outport  Port=4
  timestamp : Outport  Port=5
  wires:
  Level-2 M-file S-Function/1 -> numbers/1
  Level-2 M-file S-Function/2 -> code/1
  Level-2 M-file S-Function/3 -> parameter/1
  Level-2 M-file S-Function/4 -> Xtimes/1
  Level-2 M-file S-Function/5 -> timestamp/1
  In1/1 -> Level-2 M-file S-Function/1

== system HANcoder_STM32_Target/STM32-P405/Error Handling/Read stored error ==
  In1 : Inport
  Level-2 M-file S-Function : M-S-Function  FunctionName=sfcn_controller_error_readerror  Parameters=tsamp
  numbers : Outport
  code : Outport  Port=2
  parameter : Outport  Port=3
  Xtimes : Outport  Port=4
  timestamp : Outport  Port=5
  wires:
  In1/1 -> Level-2 M-file S-Function/1
  Level-2 M-file S-Function/5 -> timestamp/1
  Level-2 M-file S-Function/4 -> Xtimes/1
  Level-2 M-file S-Function/3 -> parameter/1
  Level-2 M-file S-Function/2 -> code/1
  Level-2 M-file S-Function/1 -> numbers/1

== system HANcoder_STM32_Target/STM32-P405/Error Handling/Search active error ==
  In1 : Inport
  In2 : Inport  Port=2
  Level-2 M-file S-Function : M-S-Function  FunctionName=sfcn_controller_error_searcherror  Parameters=tsamp
  occurrence : Outport
  timestamp : Outport  Port=2
  wires:
  In1/1 -> Level-2 M-file S-Function/1
  In2/1 -> Level-2 M-file S-Function/2
  Level-2 M-file S-Function/1 -> occurrence/1
  Level-2 M-file S-Function/2 -> timestamp/1

== system HANcoder_STM32_Target/STM32-P405/Error Handling/Search stored error ==
  In1 : Inport
  In2 : Inport  Port=2
  Level-2 M-file S-Function : M-S-Function  FunctionName=sfcn_controller_error_searcherror  Parameters=tsamp
  occurrence : Outport
  timestamp : Outport  Port=2
  wires:
  Level-2 M-file S-Function/2 -> timestamp/1
  Level-2 M-file S-Function/1 -> occurrence/1
  In2/1 -> Level-2 M-file S-Function/2
  In1/1 -> Level-2 M-file S-Function/1

== system HANcoder_STM32_Target/STM32-P405/Error Handling/Store error  ==
  Trigger : TriggerPort  VariantControl=(inherit)
  Gnd1 : Ground
  Gnd2 : Ground
  Level-2 M-file S-Function : M-S-Function  FunctionName=sfcn_controller_error_storeerror_in  Parameters=useInPorts, errorCode, parameter
  wires:
  Gnd1/1 -> Level-2 M-file S-Function/1
  Gnd2/1 -> Level-2 M-file S-Function/2

== system HANcoder_STM32_Target/STM32-P405/Error Handling/Total Errors ==
  Level-2 M-file S-Function : M-S-Function  FunctionName=sfcn_controller_error_totalerrors  Parameters=eepromString, tsamp
  Out1 : Outport
  Out2 : Outport  Port=2
  wires:
  Level-2 M-file S-Function/1 -> Out1/1
  Level-2 M-file S-Function/2 -> Out2/1

== system HANcoder_STM32_Target/STM32-P405/File Logger/File Logger Close ==
  Trigger : TriggerPort  VariantControl=(inherit)
  Level-2 M-file S-Function : M-S-Function  FunctionName=sfcn_filelogger_close

== system HANcoder_STM32_Target/STM32-P405/File Logger/File Logger Init ==
  (Re)start : TriggerPort  VariantControl=(inherit)
  Level-2 M-file S-Function : M-S-Function  FunctionName=sfcn_filelogger_init

== system HANcoder_STM32_Target/STM32-P405/File Logger/File Logger Signal ==
  In1 : Inport
  Level-2 M-file S-Function : M-S-Function  FunctionName=sfcn_filelogger_signal  Parameters=dataType
  wires:
  In1/1 -> Level-2 M-file S-Function/1

== system HANcoder_STM32_Target/STM32-P405/Memory/EEPROM ==
  Erase EEPROM : Subsystem  Tag=HANcoder_TARGET_STM32_P405  mask(Erase EEPROM){}
      mask help:
      | Function
      | ========
      | Erases all identifier values from EEPROM.
      |
      | Triggerport
      | ===========
      | Connect the port to a trigger source to execute the block only when necessary.
      mask init:
      | sfcn_eeprom_clear_mcb();
      settings: MoveFcn=drawLogos
      mask Display: fprintf('Erase EEPROM');patch([80 86 86],[8 14 2],[1 0 0]);patch([88 88 94],[14 2 8],[0 0 0.35]);
  Read from EEPROM : Subsystem  Tag=HANcoder_TARGET_STM32_P405  mask(Read from EEPROM){tsamp=-1}
      mask prompts: tsamp "Sample time"
      mask help:
      | Function
      | ========
      | Read a value from the specified EEPROM identifier.
      |
      | Inport
      | ==========
      | id:
      |   The EEPROM identifier. This input is of type UINT8 and can have a value
      |   between 0..255 to select one of the 256 supported application specific
      |   identifiers.
      |
      | Outport
      | =======
      | value:
      |   The value read from the EEPROM identifier. This output is of type UINT16.
      mask init:
      | sfcn_eeprom_read_mcb();
      settings: MoveFcn=drawLogos
      mask Display:
      | fprintf('Read from EEPROM');
      | port_label('input', 1, 'id');
      | port_label('output', 1, 'value');patch([150 156 156],[8 14 2],[1 0 0]);patch([158 158 164],[14 2 8],[0 0 0.35]);
  Save EEPROM : Subsystem  Tag=HANcoder_TARGET_STM32_P405  mask(Save EEPROM){}
      mask help:
      | Function
      | ========
      | The STM32 controller does not have dedicated EEPROM on-chip. All EEPROM
      | write, read and erase operations are therefore performed in a RAM buffer.
      | To make sure RAM buffer contents are still valid after a power-off, its
      | contents needs to be save in flash EEPROM, which is achieved with this
      | block. This is typically called during the software shutdown sequence,
      | right before power off.
      |
      | Triggerport
      | ===========
      | Connect the port to a trigger source to execute the block only when necessary.
      mask init:
      | sfcn_eeprom_save_mcb();
      settings: MoveFcn=drawLogos
      mask Display: fprintf('Save EEPROM');patch([80 86 86],[8 14 2],[1 0 0]);patch([88 88 94],[14 2 8],[0 0 0.35]);
  Write to EEPROM : Subsystem  Tag=HANcoder_TARGET_STM32_P405  mask(Write to EEPROM){tsamp=-1}
      mask prompts: tsamp "Sample time"
      mask help:
      | Function
      | ========
      | Write the value to the specified EEPROM identifier.
      |
      | Inport
      | ==========
      | id:
      |   The EEPROM identifier. This input is of type UINT8 and can have a value
      |   between 0..255 to select one of the 256 supported application specific
      |   identifiers.
      | value:
      |   The value to write to the EEPROM identifier. This input is of type UINT16.
      mask init:
      | sfcn_eeprom_write_mcb();
      settings: MoveFcn=drawLogos
      mask Display:
      | fprintf('Write to EEPROM');
      | port_label('input', 1, 'id');
      | port_label('input', 2, 'value');patch([150 156 156],[8 14 2],[1 0 0]);patch([158 158 164],[14 2 8],[0 0 0.35]);

== system HANcoder_STM32_Target/STM32-P405/PWM Outputs/PWM Duty Cycle ==
  In1 : Inport
  Level-2 M-file S-Function : M-S-Function  FunctionName=sfcn_pwmout_setduty  Parameters=tsamp
  wires:
  In1/1 -> Level-2 M-file S-Function/1
